simulink model "FMS"  (R2018b)
settings: configuration reference "FMS_config" (kept outside this file)
values from neighbouring files (symbols this model uses):
  FMS_EXPORT = Simulink.Parameter(FMS_EXPORT_VALUE)    [base_fms_init.m]    (also in base_fms_var.m; fms_model_init.m)
  FMS_PARAM = Simulink.Parameter(FMS_PARAM_VALUE)    [base_fms_init.m]    (also in base_fms_var.m; fms_model_init.m)
undefined symbols (not defined in the file or in its folder): actuator_cmd, DiscIntNeverNeededParam, mode, p_cmd, phi_cmd, psi_rate_cmd, q_cmd, r_cmd, reset, state, theta_cmd, throttle_cmd, timestamp, u_cmd, v_cmd, w_cmd
libraries: simulink x31, Rotation x2, Filter x2
(part 1 of 2)
settings Model: Creator=zouji  LastModifiedBy=zouji
settings ConfigSetRef: SourceLocation=Base Workspace

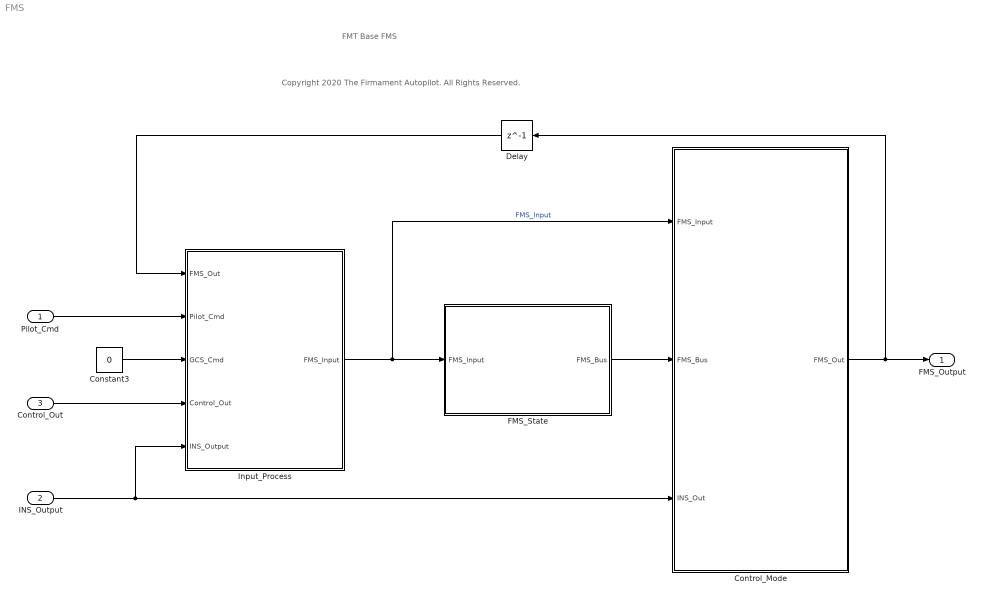
== system FMS ==
  note: FMT Base FMS
  note: Copyright 2020 The Firmament Autopilot. All Rights Reserved.
  Pilot_Cmd : Inport  OutDataTypeStr=Bus: Pilot_Cmd_Bus
  INS_Output : Inport  Port=2  OutDataTypeStr=Bus: INS_Out_Bus
  Control_Out : Inport  Port=3  OutDataTypeStr=Bus: Control_Out_Bus
  Constant3 : Constant  Value=0
  Control_Mode : Subsystem  TreatAsAtomicUnit=on
  Delay : Delay  DelayLength=1
  FMS_State : Subsystem  TreatAsAtomicUnit=on
  Input_Process : Subsystem  TreatAsAtomicUnit=on
  FMS_Output : Outport  OutDataTypeStr=Bus: FMS_Out_Bus
  wires:
  Control_Mode/1(FMS_Out) -> FMS_Output/1, Delay/1
  INS_Output/1 -> Input_Process/5(INS_Output), Control_Mode/3(INS_Out)
  Pilot_Cmd/1 -> Input_Process/2(Pilot_Cmd)
  Constant3/1 -> Input_Process/3(GCS_Cmd)
  Input_Process/1(FMS_Input) -> Control_Mode/1(FMS_Input), FMS_State/1(FMS_Input)  "FMS_Input"
  FMS_State/1(FMS_Bus) -> Control_Mode/2(FMS_Bus)
  Delay/1 -> Input_Process/1(FMS_Out)
  Control_Out/1 -> Input_Process/4(Control_Out)

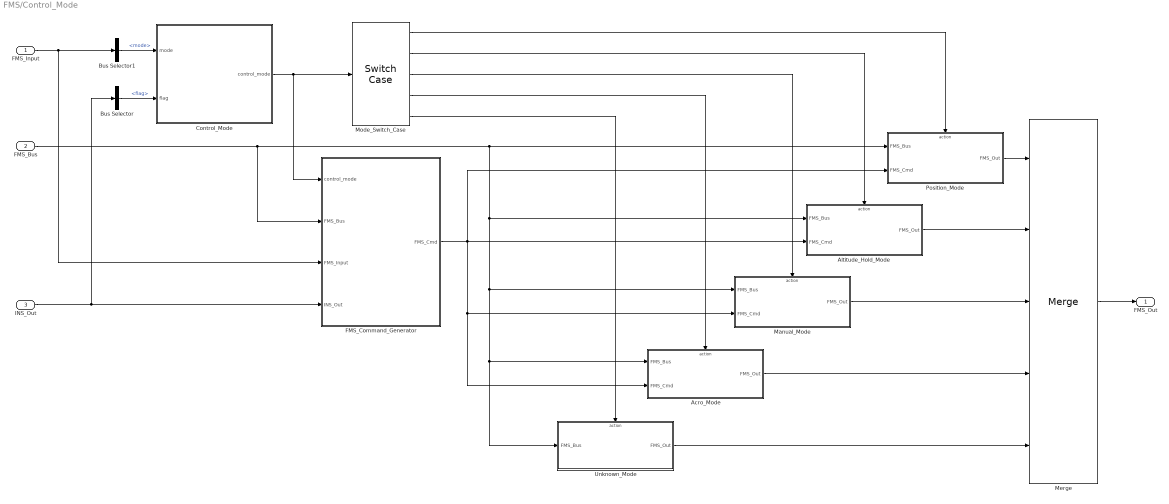
== system FMS/Control_Mode ==
  FMS_Input : Inport
  FMS_Bus : Inport  Port=2
  INS_Out : Inport  Port=3
  Acro_Mode : Subsystem  TreatAsAtomicUnit=on
  Altitude_Hold_Mode : Subsystem  TreatAsAtomicUnit=on
  Bus Selector : BusSelector  OutputSignals=flag
  Bus Selector1 : BusSelector  OutputSignals=stick_val.mode
  Control_Mode : Stateflow chart  TreatAsAtomicUnit=on
  FMS_Command_Generator : Subsystem
  Manual_Mode : Subsystem  TreatAsAtomicUnit=on
  Merge : Merge  Inputs=5
  Mode_Switch_Case : SwitchCase  CaseConditions={2,3,4,5}
  Position_Mode : Subsystem  TreatAsAtomicUnit=on
  Unknown_Mode : Subsystem  TreatAsAtomicUnit=on
  FMS_Out : Outport
  wires:
  INS_Out/1 -> Bus Selector/1, FMS_Command_Generator/4(INS_Out)
  FMS_Input/1 -> FMS_Command_Generator/3(FMS_Input), Bus Selector1/1
  Mode_Switch_Case/1 -> Position_Mode/Action
  Position_Mode/1(FMS_Out) -> Merge/1
  Mode_Switch_Case/5 -> Unknown_Mode/Action
  Bus Selector/1 -> Control_Mode/2(flag)  "<flag>"
  Merge/1 -> FMS_Out/1
  Unknown_Mode/1(FMS_Out) -> Merge/5
  FMS_Bus/1 -> Position_Mode/1(FMS_Bus), Unknown_Mode/1(FMS_Bus), Acro_Mode/1(FMS_Bus), Manual_Mode/1(FMS_Bus), Altitude_Hold_Mode/1(FMS_Bus), FMS_Command_Generator/2(FMS_Bus)
  Bus Selector1/1 -> Control_Mode/1(mode)  "<mode>"
  Control_Mode/1(control_mode) -> Mode_Switch_Case/1, FMS_Command_Generator/1(control_mode)
  Mode_Switch_Case/2 -> Altitude_Hold_Mode/Action
  Altitude_Hold_Mode/1(FMS_Out) -> Merge/2
  Mode_Switch_Case/3 -> Manual_Mode/Action
  Manual_Mode/1(FMS_Out) -> Merge/3
  Acro_Mode/1(FMS_Out) -> Merge/4
  Mode_Switch_Case/4 -> Acro_Mode/Action
  FMS_Command_Generator/1(FMS_Cmd) -> Acro_Mode/2(FMS_Cmd), Manual_Mode/2(FMS_Cmd), Altitude_Hold_Mode/2(FMS_Cmd), Position_Mode/2(FMS_Cmd)

== system FMS/FMS_State ==
  FMS_Input : Inport
  Bus Assignment : BusAssignment  AssignedSignals=actuator_cmd,state,reset,timestamp
  Bus Selector : BusSelector  OutputSignals=stick_val.stick_throttle_raw,event_cmd.arm_event,event_cmd.disarm_event,event_cmd.force_disarm_event,state_cmd.test_motor_state
  Compare To Constant : simulink/Logic and Bit Operations/Compare To Constant  relop=<  const=2  OutDataTypeStr=uint8
  Constant : Constant  Value=0  OutDataTypeStr=Bus: FMS_Out_Bus
  State_Management : Stateflow chart  TreatAsAtomicUnit=on
  expand_pwm : Subsystem
  timestamp : Subsystem  mask{sample_time=FMS_EXPORT.period}
      mask prompts: sample_time "sample time (ms)"
  FMS_Bus : Outport
  wires:
  Constant/1 -> Bus Assignment/1
  Bus Assignment/1 -> FMS_Bus/1
  FMS_Input/1 -> Bus Selector/1
  State_Management/1(PWM_Cmd) -> expand_pwm/1(pwm_in)
  expand_pwm/1(pwm_out) -> Bus Assignment/2
  Compare To Constant/1 -> Bus Assignment/4
  timestamp/1(timestamp_ms) -> Bus Assignment/5
  Bus Selector/1 -> State_Management/1(stick_throttle)  "<stick_throttle_raw>"
  Bus Selector/2 -> State_Management/2(arm_event)  "<arm_event>"
  Bus Selector/3 -> State_Management/3(disarm_event)  "<disarm_event>"
  Bus Selector/4 -> State_Management/4(force_disarm_event)  "<force_disarm_event>"
  Bus Selector/5 -> State_Management/5(test_motor_state)  "<test_motor_state>"
  State_Management/2(State) -> Compare To Constant/1, Bus Assignment/3

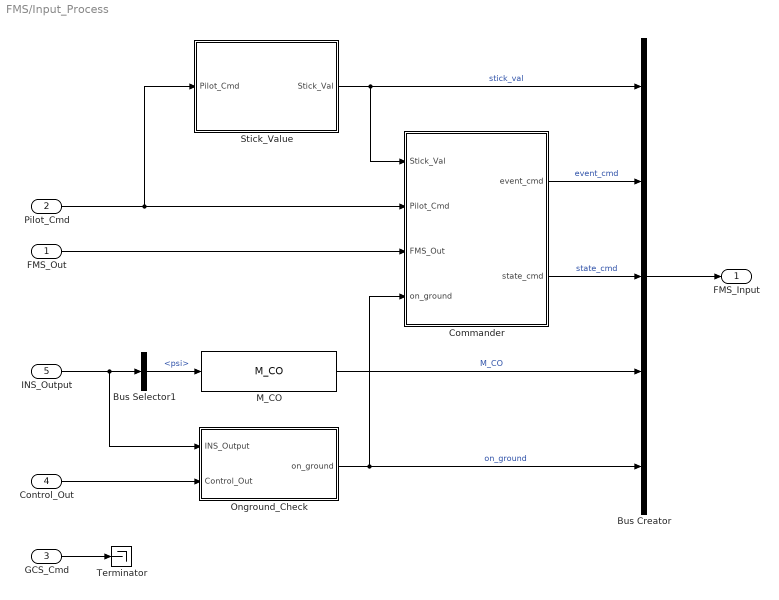
== system FMS/Input_Process ==
  FMS_Out : Inport
  Pilot_Cmd : Inport  Port=2
  GCS_Cmd : Inport  Port=3
  Control_Out : Inport  Port=4
  INS_Output : Inport  Port=5
  Bus Creator : BusCreator  Inputs=5
  Bus Selector1 : BusSelector  OutputSignals=psi
  Commander : Subsystem
  M_CO : Rotation/M_CO  SystemSampleTime=-1
  Onground_Check : Subsystem
  Stick_Value : Subsystem
  Terminator : Terminator
  FMS_Input : Outport
  wires:
  GCS_Cmd/1 -> Terminator/1
  Pilot_Cmd/1 -> Stick_Value/1(Pilot_Cmd), Commander/2(Pilot_Cmd)
  Bus Creator/1 -> FMS_Input/1
  INS_Output/1 -> Onground_Check/1(INS_Output), Bus Selector1/1
  Bus Selector1/1 -> M_CO/1  "<psi>"
  M_CO/1 -> Bus Creator/4  "M_CO"
  Commander/1(event_cmd) -> Bus Creator/2  "event_cmd"
  Commander/2(state_cmd) -> Bus Creator/3  "state_cmd"
  Stick_Value/1(Stick_Val) -> Commander/1(Stick_Val), Bus Creator/1  "stick_val"
  FMS_Out/1 -> Commander/3(FMS_Out)
  Control_Out/1 -> Onground_Check/2(Control_Out)
  Onground_Check/1(on_ground) -> Commander/4(on_ground), Bus Creator/5  "on_ground"

== system FMS/Control_Mode/Acro_Mode ==
  FMS_Bus : Inport
  FMS_Cmd : Inport  Port=2
  Action Port : ActionPort  InitializeStates=reset  ActionType=case
  Bus Assignment : BusAssignment  AssignedSignals=mode,throttle_cmd,p_cmd,q_cmd,r_cmd
  Bus Selector : BusSelector  OutputSignals=throttle_cmd,p_cmd,q_cmd,r_cmd
  Constant : Constant  Value=5  OutDataTypeStr=Inherit: Inherit via back propagation
  FMS_Out : Outport
  wires:
  Bus Assignment/1 -> FMS_Out/1
  Constant/1 -> Bus Assignment/2
  FMS_Bus/1 -> Bus Assignment/1
  Bus Selector/1 -> Bus Assignment/3  "<throttle_cmd>"
  Bus Selector/2 -> Bus Assignment/4  "<p_cmd>"
  Bus Selector/3 -> Bus Assignment/5  "<q_cmd>"
  Bus Selector/4 -> Bus Assignment/6  "<r_cmd>"
  FMS_Cmd/1 -> Bus Selector/1

== system FMS/Control_Mode/Altitude_Hold_Mode ==
  FMS_Bus : Inport
  FMS_Cmd : Inport  Port=2
  Action Port : ActionPort  InitializeStates=reset  ActionType=case
  Bus Assignment : BusAssignment  AssignedSignals=mode,phi_cmd,theta_cmd,w_cmd,psi_rate_cmd
  Bus Selector : BusSelector  OutputSignals=phi_cmd,thera_cmd,w_cmd,psi_rate_cmd
  alt_hold_mode : Constant  Value=3  OutDataTypeStr=Inherit: Inherit via back propagation
  FMS_Out : Outport
  wires:
  FMS_Bus/1 -> Bus Assignment/1
  alt_hold_mode/1 -> Bus Assignment/2
  FMS_Cmd/1 -> Bus Selector/1
  Bus Assignment/1 -> FMS_Out/1
  Bus Selector/3 -> Bus Assignment/5  "<w_cmd>"
  Bus Selector/4 -> Bus Assignment/6  "<psi_rate_cmd>"
  Bus Selector/1 -> Bus Assignment/3  "<phi_cmd>"
  Bus Selector/2 -> Bus Assignment/4  "<thera_cmd>"

== system FMS/Control_Mode/FMS_Command_Generator ==
  control_mode : Inport
  FMS_Bus : Inport  Port=2
  FMS_Input : Inport  Port=3
  INS_Out : Inport  Port=4
  Angel_Rate_Command : Subsystem
  Attitude_Command : Subsystem
  Bus Creator : BusCreator  Inputs=10
  Psi_Rate_Command : Subsystem
  Throttle_Command : Subsystem
  Velocity_Command : Subsystem
  FMS_Cmd : Outport
  wires:
  FMS_Input/1 -> Attitude_Command/1(FMS_Input), Velocity_Command/2(FMS_Input), Throttle_Command/1(FMS_Input), Angel_Rate_Command/1(FMS_Input), Psi_Rate_Command/1(FMS_Input)
  INS_Out/1 -> Psi_Rate_Command/2(INS_Out), Velocity_Command/3(INS_Out)
  FMS_Bus/1 -> Psi_Rate_Command/3(FMS_Bus), Velocity_Command/4(FMS_Bus)
  Attitude_Command/1(phi_cmd_rad) -> Bus Creator/1  "phi_cmd"
  Attitude_Command/2(theta_cmd_rad) -> Bus Creator/2  "thera_cmd"
  Psi_Rate_Command/1(psi_rate_cmd_radPs) -> Bus Creator/3  "psi_rate_cmd"
  Velocity_Command/1(vel_u_cmd_C_mPs) -> Bus Creator/4  "u_cmd"
  Velocity_Command/2(vel_v_cmd_C_mPs) -> Bus Creator/5  "v_cmd"
  Velocity_Command/3(vel_w_cmd_C_mPs) -> Bus Creator/6  "w_cmd"
  Throttle_Command/1(throttle_cmd) -> Bus Creator/7  "throttle_cmd"
  Angel_Rate_Command/1(p_cmd_radPs) -> Bus Creator/8  "p_cmd"
  Angel_Rate_Command/2(q_cmd_radPs) -> Bus Creator/9  "q_cmd"
  Angel_Rate_Command/3(r_cmd_radPs) -> Bus Creator/10  "r_cmd"
  Bus Creator/1 -> FMS_Cmd/1
  control_mode/1 -> Velocity_Command/1(control_mode), Psi_Rate_Command/4(control_mode)

== system FMS/Control_Mode/Manual_Mode ==
  FMS_Bus : Inport
  FMS_Cmd : Inport  Port=2
  Action Port : ActionPort  InitializeStates=reset  ActionType=case
  Bus Assignment : BusAssignment  AssignedSignals=mode,throttle_cmd,phi_cmd,theta_cmd,psi_rate_cmd
  Bus Selector : BusSelector  OutputSignals=throttle_cmd,phi_cmd,thera_cmd,psi_rate_cmd
  manual_mode : Constant  Value=4  OutDataTypeStr=Inherit: Inherit via back propagation
  FMS_Out : Outport
  wires:
  Bus Assignment/1 -> FMS_Out/1
  FMS_Cmd/1 -> Bus Selector/1
  manual_mode/1 -> Bus Assignment/2
  FMS_Bus/1 -> Bus Assignment/1
  Bus Selector/1 -> Bus Assignment/3  "<throttle_cmd>"
  Bus Selector/2 -> Bus Assignment/4  "<phi_cmd>"
  Bus Selector/3 -> Bus Assignment/5  "<thera_cmd>"
  Bus Selector/4 -> Bus Assignment/6  "<psi_rate_cmd>"

== system FMS/Control_Mode/Position_Mode ==
  FMS_Bus : Inport
  FMS_Cmd : Inport  Port=2
  Action Port : ActionPort  InitializeStates=reset  ActionType=case
  Bus Assignment : BusAssignment  AssignedSignals=mode,u_cmd,v_cmd,w_cmd,psi_rate_cmd
  Bus Selector : BusSelector  OutputSignals=u_cmd,v_cmd,w_cmd,psi_rate_cmd
  position_mode : Constant  Value=2  OutDataTypeStr=Inherit: Inherit via back propagation
  FMS_Out : Outport
  wires:
  FMS_Bus/1 -> Bus Assignment/1
  position_mode/1 -> Bus Assignment/2
  Bus Assignment/1 -> FMS_Out/1
  Bus Selector/1 -> Bus Assignment/3  "<u_cmd>"
  Bus Selector/2 -> Bus Assignment/4  "<v_cmd>"
  Bus Selector/3 -> Bus Assignment/5  "<w_cmd>"
  Bus Selector/4 -> Bus Assignment/6  "<psi_rate_cmd>"
  FMS_Cmd/1 -> Bus Selector/1

== system FMS/Control_Mode/Unknown_Mode ==
  FMS_Bus : Inport
  Action Port : ActionPort  InitializeStates=reset  ActionType=default
  Bus Assignment : BusAssignment  AssignedSignals=mode,reset
  Constant1 : Constant  Value=0  OutDataTypeStr=Inherit: Inherit via back propagation
  Constant2 : Constant  OutDataTypeStr=Inherit: Inherit via back propagation
  FMS_Out : Outport
  wires:
  Bus Assignment/1 -> FMS_Out/1
  FMS_Bus/1 -> Bus Assignment/1
  Constant1/1 -> Bus Assignment/2
  Constant2/1 -> Bus Assignment/3

== system FMS/FMS_State/expand_pwm ==
  pwm_in : Inport
  Multiply : Product  OutDataTypeStr=uint16
  One : Constant  Value=ones(16,1)  OutDataTypeStr=uint16
  pwm_out : Outport
  wires:
  pwm_in/1 -> Multiply/2
  One/1 -> Multiply/1
  Multiply/1 -> pwm_out/1

== system FMS/FMS_State/timestamp ==
  Constant : Constant  Value=sample_time  OutDataTypeStr=uint32
  Data Type Conversion : DataTypeConversion  OutDataTypeStr=uint32
  Discrete-Time Integrator : DiscreteIntegrator  IntegratorMethod=Accumulation: Forward Euler  SampleTime=-1  ICPrevOutput=DiscIntNeverNeededParam  ICPrevScaledInput=DiscIntNeverNeededParam
  timestamp_ms : Outport
  wires:
  Discrete-Time Integrator/1 -> Data Type Conversion/1
  Constant/1 -> Discrete-Time Integrator/1
  Data Type Conversion/1 -> timestamp_ms/1

== system FMS/Input_Process/Commander ==
  Stick_Val : Inport
  Pilot_Cmd : Inport  Port=2
  FMS_Out : Inport  Port=3
  on_ground : Inport  Port=4
  Event_Commander : Subsystem
  State_Commander : Subsystem
  event_cmd : Outport
  state_cmd : Outport  Port=2
  wires:
  Pilot_Cmd/1 -> State_Commander/1(Pilot_Cmd), Event_Commander/3(Pilot_Cmd)
  Event_Commander/1(Event_Cmd) -> event_cmd/1
  FMS_Out/1 -> Event_Commander/2(FMS_Out)
  Stick_Val/1 -> Event_Commander/1(Stick_Val)
  on_ground/1 -> Event_Commander/4(on_ground)
  State_Commander/1(State_Cmd) -> state_cmd/1

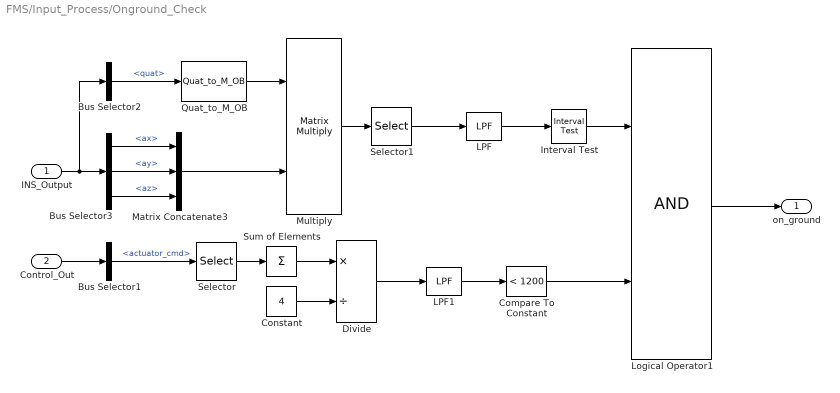
== system FMS/Input_Process/Onground_Check ==
  INS_Output : Inport
  Control_Out : Inport  Port=2
  Bus Selector1 : BusSelector  OutputSignals=actuator_cmd
  Bus Selector2 : BusSelector  OutputSignals=quat
  Bus Selector3 : BusSelector  OutputSignals=ax,ay,az
  Compare To Constant : simulink/Logic and Bit Operations/Compare To Constant  relop=<  const=1200  OutDataTypeStr=boolean
  Constant : Constant  Value=4  OutDataTypeStr=uint16
  Divide : Product  Inputs=*/
  Interval Test : simulink/Logic and Bit Operations/Interval Test  IntervalClosedRight=on  uplimit=single(-9.806+1)  IntervalClosedLeft=on  lowlimit=single(-9.806-1)  OutDataTypeStr=boolean
  LPF : Filter/LPF  T=0.5
  LPF1 : Filter/LPF  T=0.1
  Logical Operator1 : Logic  AllPortsSameDT=off  OutDataTypeStr=boolean
  Matrix Concatenate3 : Concatenate  NumInputs=3  ConcatenateDimension=2
  Multiply : Product  Multiplication=Matrix(*)
  Quat_to_M_OB : Rotation/Quat_to_M_OB  SystemSampleTime=-1
  Selector : Selector  InputPortWidth=16  IndexOptions=Index vector (dialog)  Indices=[1:4]  OutputSizes=1
  Selector1 : Selector  InputPortWidth=3  IndexOptions=Index vector (dialog)  Indices=3  OutputSizes=1
  Sum of Elements : Sum  Inputs=+
  on_ground : Outport
  wires:
  Multiply/1 -> Selector1/1
  Quat_to_M_OB/1 -> Multiply/1
  Bus Selector3/2 -> Matrix Concatenate3/2  "<ay>"
  Compare To Constant/1 -> Logical Operator1/2
  Bus Selector3/3 -> Matrix Concatenate3/3  "<az>"
  Matrix Concatenate3/1 -> Multiply/2
  Bus Selector1/1 -> Selector/1  "<actuator_cmd>"
  Bus Selector3/1 -> Matrix Concatenate3/1  "<ax>"
  Bus Selector2/1 -> Quat_to_M_OB/1  "<quat>"
  Selector/1 -> Sum of Elements/1
  INS_Output/1 -> Bus Selector2/1, Bus Selector3/1
  Logical Operator1/1 -> on_ground/1
  Control_Out/1 -> Bus Selector1/1
  Selector1/1 -> LPF/1
  Interval Test/1 -> Logical Operator1/1
  Sum of Elements/1 -> Divide/1
  Constant/1 -> Divide/2
  Divide/1 -> LPF1/1
  LPF/1 -> Interval Test/1
  LPF1/1 -> Compare To Constant/1

== system FMS/Input_Process/Stick_Value ==
  Pilot_Cmd : Inport
  Bus Creator : BusCreator  Inputs=9
  Bus Selector : BusSelector  OutputSignals=ls_lr,ls_ud,rs_lr,rs_ud,mode
  Dead_Zone : Subsystem  mask{len=FMS_PARAM.YAW_DZ}
      mask prompts: len "Zone Half Length"
  Dead_Zone1 : Subsystem  mask{len=FMS_PARAM.THROTTLE_DZ}
      mask prompts: len "Zone Half Length"
  Dead_Zone2 : Subsystem  mask{len=FMS_PARAM.ROLL_DZ}
      mask prompts: len "Zone Half Length"
  Dead_Zone3 : Subsystem  mask{len=FMS_PARAM.PITCH_DZ}
      mask prompts: len "Zone Half Length"
  Saturation{,1..3} (4 alike) : Saturate  UpperLimit=1  LowerLimit=-1
  Signal Copy4 : SignalConversion  OverrideOpt=off
  Stick_Val : Outport
  wires:
  Saturation/1 -> Bus Creator/2, Dead_Zone/1(in)  "stick_yaw_raw"
  Bus Selector/2 -> Saturation1/1  "<ls_ud>"
  Bus Selector/1 -> Saturation/1  "<ls_lr>"
  Saturation2/1 -> Bus Creator/6, Dead_Zone2/1(in)  "stick_roll_raw"
  Saturation1/1 -> Bus Creator/4, Dead_Zone1/1(in)  "stick_throttle_raw"
  Saturation3/1 -> Bus Creator/8, Dead_Zone3/1(in)  "stick_pitch_raw"
  Bus Selector/5 -> Signal Copy4/1  "<mode>"
  Bus Selector/3 -> Saturation2/1  "<rs_lr>"
  Bus Selector/4 -> Saturation3/1  "<rs_ud>"
  Dead_Zone/1(out) -> Bus Creator/1  "stick_yaw"
  Pilot_Cmd/1 -> Bus Selector/1
  Dead_Zone1/1(out) -> Bus Creator/3  "stick_throttle"
  Dead_Zone2/1(out) -> Bus Creator/5  "stick_roll"
  Dead_Zone3/1(out) -> Bus Creator/7  "stick_pitch"
  Signal Copy4/1 -> Bus Creator/9  "mode"
  Bus Creator/1 -> Stick_Val/1

== system FMS/Control_Mode/FMS_Command_Generator/Angel_Rate_Command ==
  FMS_Input : Inport
  Bus Selector : BusSelector  OutputSignals=stick_val.stick_roll_raw,stick_val.stick_pitch_raw,stick_val.stick_yaw_raw
  Gain : Gain  Gain=pi/3  OutDataTypeStr=Inherit: Same as input
  Gain1 : Gain  Gain=-pi/3  OutDataTypeStr=Inherit: Same as input
  Gain2 : Gain  Gain=pi/3  OutDataTypeStr=Inherit: Same as input
  p_cmd_radPs : Outport
  q_cmd_radPs : Outport  Port=2
  r_cmd_radPs : Outport  Port=3
  wires:
  Bus Selector/2 -> Gain1/1  "<stick_pitch_raw>"
  Bus Selector/1 -> Gain/1  "<stick_roll_raw>"
  FMS_Input/1 -> Bus Selector/1
  Gain/1 -> p_cmd_radPs/1
  Gain1/1 -> q_cmd_radPs/1
  Bus Selector/3 -> Gain2/1  "<stick_yaw_raw>"
  Gain2/1 -> r_cmd_radPs/1

== system FMS/Control_Mode/FMS_Command_Generator/Attitude_Command ==
  FMS_Input : Inport
  Bus Selector : BusSelector  OutputSignals=stick_val.stick_roll,stick_val.stick_pitch
  Gain : Gain  Gain=FMS_PARAM.ROLL_PITCH_LIM
  Gain1 : Gain  Gain=-FMS_PARAM.ROLL_PITCH_LIM
  Phi_CMD_TD : Subsystem
  Thera_CMD_TD : Subsystem
  phi_cmd_rad : Outport
  theta_cmd_rad : Outport  Port=2
  wires:
  Gain/1 -> Phi_CMD_TD/1(v)
  FMS_Input/1 -> Bus Selector/1
  Bus Selector/1 -> Gain/1  "<stick_roll>"
  Bus Selector/2 -> Gain1/1  "<stick_pitch>"
  Gain1/1 -> Thera_CMD_TD/1(v)
  Phi_CMD_TD/1(v1) -> phi_cmd_rad/1
  Thera_CMD_TD/1(v1) -> theta_cmd_rad/1

== system FMS/Control_Mode/FMS_Command_Generator/Psi_Rate_Command ==
  FMS_Input : Inport
  INS_Out : Inport  Port=2
  FMS_Bus : Inport  Port=3
  control_mode : Inport  Port=4
  Bus Selector : BusSelector  OutputSignals=state
  Motion_Check : Subsystem
  Psi_Rate_Commander : Subsystem
  Update : Subsystem
  psi_rate_cmd_radPs : Outport
  wires:
  INS_Out/1 -> Motion_Check/2(INS_Out), Psi_Rate_Commander/4(INS_Out)
  FMS_Input/1 -> Motion_Check/1(FMS_Input), Psi_Rate_Commander/2(FMS_Input)
  FMS_Bus/1 -> Bus Selector/1
  Motion_Check/1(psi_motion_state) -> Psi_Rate_Commander/3(motion_state), Update/3(motion_state)  "psi_motion_state"
  Psi_Rate_Commander/1(psi_rate_cmd_radPs) -> psi_rate_cmd_radPs/1
  Update/1(update) -> Psi_Rate_Commander/1(update)
  control_mode/1 -> Update/2(control_mode)
  Bus Selector/1 -> Update/1(state)  "<state>"

== system FMS/Control_Mode/FMS_Command_Generator/Throttle_Command ==
  FMS_Input : Inport
  Add : Sum
  Bus Selector : BusSelector  OutputSignals=stick_val.stick_throttle_raw
  Constant : Constant  OutDataTypeStr=single
  Constant1 : Constant  Value=1000  OutDataTypeStr=uint32
  Gain : Gain  Gain=500  OutDataTypeStr=uint32
  Saturation : Saturate  UpperLimit=2  LowerLimit=0
  Sum : Sum  Inputs=|++
  throttle_cmd : Outport
  wires:
  FMS_Input/1 -> Bus Selector/1
  Gain/1 -> Add/1
  Bus Selector/1 -> Sum/1  "<stick_throttle_raw>"
  Add/1 -> throttle_cmd/1
  Constant/1 -> Sum/2
  Sum/1 -> Saturation/1
  Constant1/1 -> Add/2
  Saturation/1 -> Gain/1

== system FMS/Control_Mode/FMS_Command_Generator/Velocity_Command ==
  control_mode : Inport
  FMS_Input : Inport  Port=2
  INS_Out : Inport  Port=3
  FMS_Bus : Inport  Port=4
  Bus Selector : BusSelector  OutputSignals=state
  Demux : Demux  Outputs=3
  Motion_Check : Subsystem
  Update : Subsystem
  Velocity_Commander : Subsystem
  vel_u_cmd_C_mPs : Outport
  vel_v_cmd_C_mPs : Outport  Port=2
  vel_w_cmd_C_mPs : Outport  Port=3
  wires:
  Velocity_Commander/1(vel_cmd_C_mPs) -> Demux/1
  FMS_Input/1 -> Motion_Check/1(FMS_Input), Velocity_Commander/1(FMS_Input)
  INS_Out/1 -> Motion_Check/2(INS_Out), Velocity_Commander/4(INS_Out)
  Motion_Check/1(pos_motion_state) -> Update/3(motion_state), Velocity_Commander/3(motion_state)  "pos_motion_state"
  Demux/1 -> vel_u_cmd_C_mPs/1
  Demux/2 -> vel_v_cmd_C_mPs/1
  Demux/3 -> vel_w_cmd_C_mPs/1
  FMS_Bus/1 -> Bus Selector/1
  control_mode/1 -> Update/1(control_mode)
  Bus Selector/1 -> Update/2(state)  "<state>"
  Update/1(update) -> Velocity_Commander/2(update)  "update_pos"

== system FMS/Input_Process/Commander/Event_Commander ==
  Stick_Val : Inport
  FMS_Out : Inport  Port=2
  Pilot_Cmd : Inport  Port=3
  on_ground : Inport  Port=4
  Arm_Disarm_Event : Subsystem
  Bus Creator : BusCreator  Inputs=3
  Bus Selector2 : BusSelector  OutputSignals=cmd_1
  Compare To Constant : simulink/Logic and Bit Operations/Compare To Constant  relop===  const=1000  OutDataTypeStr=boolean
  Detect Increase : simulink/Logic and Bit Operations/Detect Increase  vinit=0.0  OutDataTypeStr=boolean
  Event_Cmd : Outport
  wires:
  Pilot_Cmd/1 -> Bus Selector2/1
  Bus Selector2/1 -> Compare To Constant/1  "<cmd_1>"
  Compare To Constant/1 -> Detect Increase/1
  Detect Increase/1 -> Bus Creator/3  "force_disarm_event"
  Bus Creator/1 -> Event_Cmd/1
  FMS_Out/1 -> Arm_Disarm_Event/2(FMS_Out)
  Stick_Val/1 -> Arm_Disarm_Event/1(Stick_Val)
  on_ground/1 -> Arm_Disarm_Event/3(on_ground)
  Arm_Disarm_Event/1(arm_event) -> Bus Creator/1  "arm_event"
  Arm_Disarm_Event/2(disarm_event) -> Bus Creator/2  "disarm_event"

== system FMS/Input_Process/Commander/State_Commander ==
  Pilot_Cmd : Inport
  Bus Creator1 : BusCreator  Inputs=1
  Bus Selector1 : BusSelector  OutputSignals=cmd_2
  Compare To Constant3 : simulink/Logic and Bit Operations/Compare To Constant  relop===  const=2000  OutDataTypeStr=boolean
  State_Cmd : Outport
  wires:
  Bus Selector1/1 -> Compare To Constant3/1  "<cmd_2>"
  Compare To Constant3/1 -> Bus Creator1/1  "test_motor_state"
  Pilot_Cmd/1 -> Bus Selector1/1
  Bus Creator1/1 -> State_Cmd/1

== system FMS/Input_Process/Stick_Value/Dead_Zone ==
  in : Inport
  Add : Sum
  Constant : Constant  Value=len  OutDataTypeStr=single
  Dead Zone : DeadZone  LowerValue=-len  UpperValue=len  SaturateOnIntegerOverflow=on
  Multiply : Product
  Sign : Signum
  out : Outport
  wires:
  in/1 -> Dead Zone/1
  Dead Zone/1 -> Sign/1, Add/1
  Sign/1 -> Multiply/1
  Constant/1 -> Multiply/2
  Multiply/1 -> Add/2
  Add/1 -> out/1

== system FMS/Input_Process/Stick_Value/Dead_Zone1 ==
  in : Inport
  Add : Sum
  Constant : Constant  Value=len  OutDataTypeStr=single
  Dead Zone : DeadZone  LowerValue=-len  UpperValue=len  SaturateOnIntegerOverflow=on
  Multiply : Product
  Sign : Signum
  out : Outport
  wires:
  Add/1 -> out/1
  Multiply/1 -> Add/2
  Constant/1 -> Multiply/2
  Sign/1 -> Multiply/1
  Dead Zone/1 -> Add/1, Sign/1
  in/1 -> Dead Zone/1

== system FMS/Input_Process/Stick_Value/Dead_Zone2 ==
  in : Inport
  Add : Sum
  Constant : Constant  Value=len  OutDataTypeStr=single
  Dead Zone : DeadZone  LowerValue=-len  UpperValue=len  SaturateOnIntegerOverflow=on
  Multiply : Product
  Sign : Signum
  out : Outport
  wires:
  in/1 -> Dead Zone/1
  Dead Zone/1 -> Sign/1, Add/1
  Sign/1 -> Multiply/1
  Constant/1 -> Multiply/2
  Multiply/1 -> Add/2
  Add/1 -> out/1

== system FMS/Input_Process/Stick_Value/Dead_Zone3 ==
  in : Inport
  Add : Sum
  Constant : Constant  Value=len  OutDataTypeStr=single
  Dead Zone : DeadZone  LowerValue=-len  UpperValue=len  SaturateOnIntegerOverflow=on
  Multiply : Product
  Sign : Signum
  out : Outport
  wires:
  Add/1 -> out/1
  Multiply/1 -> Add/2
  Constant/1 -> Multiply/2
  Sign/1 -> Multiply/1
  Dead Zone/1 -> Add/1, Sign/1
  in/1 -> Dead Zone/1

== system FMS/Control_Mode/FMS_Command_Generator/Attitude_Command/Phi_CMD_TD ==
  v : Inport
  Integrator : DiscreteIntegrator  SampleTime=-1  ICPrevOutput=DiscIntNeverNeededParam  ICPrevScaledInput=DiscIntNeverNeededParam
  Integrator1 : DiscreteIntegrator  SampleTime=-1  ICPrevOutput=DiscIntNeverNeededParam  ICPrevScaledInput=DiscIntNeverNeededParam
  Subtract : Sum  Inputs=+-
  "fhan " : Subsystem  mask{r0=4*pi, h0=0.04}
      mask DialogControl ParameterGroupVar Prompt: fhan(v1,v2,r0,h0)
  v1 : Outport
  wires:
  Integrator1/1 -> v1/1, Subtract/1
  v/1 -> Subtract/2
  Integrator/1 -> "fhan "/2(v2), Integrator1/1  "v2"
  Subtract/1 -> "fhan "/1(v1)
  "fhan "/1(fhan) -> Integrator/1

== system FMS/Control_Mode/FMS_Command_Generator/Attitude_Command/Thera_CMD_TD ==
  v : Inport
  Integrator : DiscreteIntegrator  SampleTime=-1  ICPrevOutput=DiscIntNeverNeededParam  ICPrevScaledInput=DiscIntNeverNeededParam
  Integrator1 : DiscreteIntegrator  SampleTime=-1  ICPrevOutput=DiscIntNeverNeededParam  ICPrevScaledInput=DiscIntNeverNeededParam
  Subtract : Sum  Inputs=+-
  "fhan " : Subsystem  mask{r0=4*pi, h0=0.04}
      mask DialogControl ParameterGroupVar Prompt: fhan(v1,v2,r0,h0)
  v1 : Outport
  wires:
  "fhan "/1(fhan) -> Integrator/1
  Subtract/1 -> "fhan "/1(v1)
  Integrator/1 -> "fhan "/2(v2), Integrator1/1  "v2"
  v/1 -> Subtract/2
  Integrator1/1 -> Subtract/1, v1/1

== system FMS/Control_Mode/FMS_Command_Generator/Psi_Rate_Command/Motion_Check ==
  FMS_Input : Inport
  INS_Out : Inport  Port=2
  Motion_State : Stateflow chart  TreatAsAtomicUnit=on
  heading_rate : Subsystem
  move_check : Subsystem
  psi_motion_state : Outport
  wires:
  heading_rate/1(heading_rate) -> Motion_State/2(heading_rate)
  Motion_State/1(state) -> psi_motion_state/1
  FMS_Input/1 -> move_check/1(FMS_Input)
  move_check/1(move_request) -> Motion_State/1(move_cmd)
  INS_Out/1 -> heading_rate/1(INS_Out)

== system FMS/Control_Mode/FMS_Command_Generator/Psi_Rate_Command/Psi_Rate_Commander ==
  update : Inport
  FMS_Input : Inport  Port=2
  motion_state : Inport  Port=3
  INS_Out : Inport  Port=4
  Compare To Constant : simulink/Logic and Bit Operations/Compare To Constant  relop===  const=2  OutDataTypeStr=boolean
  Heading_Control : Subsystem
  Motion_Heading_Rate : Subsystem
  Saturation : Saturate  UpperLimit=FMS_PARAM.YAW_RATE_LIM  LowerLimit=-FMS_PARAM.YAW_RATE_LIM
  Switch : Switch  Criteria=u2 > Threshold
  TD : Subsystem
  psi_rate_cmd_radPs : Outport
  wires:
  Compare To Constant/1 -> Switch/2
  motion_state/1 -> Motion_Heading_Rate/1(motion_state), Compare To Constant/1
  Heading_Control/1(psi_rate_cmd_radPs) -> Switch/1
  Motion_Heading_Rate/1(psi_rate_cmd_radPs) -> Switch/3
  INS_Out/1 -> Heading_Control/2(INS_Out)
  FMS_Input/1 -> Motion_Heading_Rate/2(FMS_Input)
  Switch/1 -> Saturation/1
  Saturation/1 -> TD/1(v)
  TD/1(v1) -> psi_rate_cmd_radPs/1
  update/1 -> Heading_Control/1(update)

== system FMS/Control_Mode/FMS_Command_Generator/Psi_Rate_Command/Update ==
  state : Inport
  control_mode : Inport  Port=2
  motion_state : Inport  Port=3
  Compare To Constant1 : simulink/Logic and Bit Operations/Compare To Constant  relop=>=  const=1  OutDataTypeStr=boolean
  Compare To Constant2 : simulink/Logic and Bit Operations/Compare To Constant  relop=<=  const=4  OutDataTypeStr=boolean
  Compare To Constant3 : simulink/Logic and Bit Operations/Compare To Constant  relop===  const=2  OutDataTypeStr=boolean
  Compare To Constant4 : simulink/Logic and Bit Operations/Compare To Constant  relop===  const=2  OutDataTypeStr=boolean
  Detect Increase1 : simulink/Logic and Bit Operations/Detect Increase  vinit=0.0  OutDataTypeStr=boolean
  Detect Increase2 : simulink/Logic and Bit Operations/Detect Increase  vinit=0.0  OutDataTypeStr=boolean
  Detect Increase3 : simulink/Logic and Bit Operations/Detect Increase  vinit=0.0  OutDataTypeStr=boolean
  Logical Operator1 : Logic  Operator=OR  Inputs=3  AllPortsSameDT=off  OutDataTypeStr=boolean
  Logical Operator2 : Logic  Operator=OR  AllPortsSameDT=off  OutDataTypeStr=boolean
  update : Outport
  wires:
  state/1 -> Compare To Constant3/1
  Compare To Constant4/1 -> Detect Increase3/1
  Compare To Constant3/1 -> Detect Increase2/1
  Detect Increase2/1 -> Logical Operator1/2
  motion_state/1 -> Compare To Constant4/1
  Logical Operator1/1 -> update/1
  Detect Increase3/1 -> Logical Operator1/1
  control_mode/1 -> Compare To Constant2/1, Compare To Constant1/1
  Compare To Constant1/1 -> Logical Operator2/1
  Compare To Constant2/1 -> Logical Operator2/2
  Logical Operator2/1 -> Detect Increase1/1
  Detect Increase1/1 -> Logical Operator1/3

== system FMS/Control_Mode/FMS_Command_Generator/Velocity_Command/Motion_Check ==
  FMS_Input : Inport
  INS_Out : Inport  Port=2
  Motion_State : Subsystem
  line_speed : Subsystem
  move_check : Subsystem
  pos_motion_state : Outport
  wires:
  INS_Out/1 -> line_speed/1(INS_Out)
  move_check/1(move_request) -> Motion_State/1(move_request)
  Motion_State/1(pos_motion_state) -> pos_motion_state/1
  FMS_Input/1 -> move_check/1(FMS_Input)
  line_speed/1(line_speed) -> Motion_State/2(line_speed)

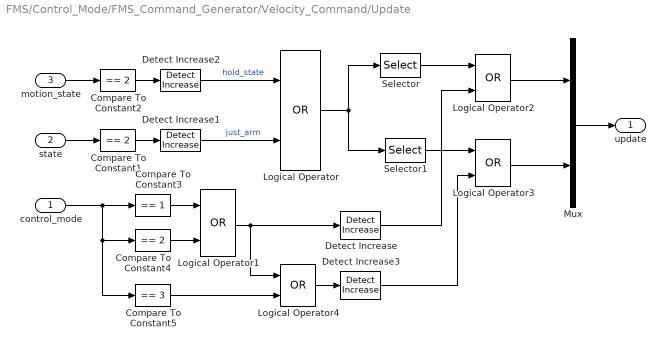
== system FMS/Control_Mode/FMS_Command_Generator/Velocity_Command/Update ==
  control_mode : Inport
  state : Inport  Port=2
  motion_state : Inport  Port=3
  Compare To Constant1 : simulink/Logic and Bit Operations/Compare To Constant  relop===  const=2  OutDataTypeStr=boolean
  Compare To Constant2 : simulink/Logic and Bit Operations/Compare To Constant  relop===  const=2  OutDataTypeStr=boolean
  Compare To Constant3 : simulink/Logic and Bit Operations/Compare To Constant  relop===  const=1  OutDataTypeStr=boolean
  Compare To Constant4 : simulink/Logic and Bit Operations/Compare To Constant  relop===  const=2  OutDataTypeStr=boolean
  Compare To Constant5 : simulink/Logic and Bit Operations/Compare To Constant  relop===  const=3  OutDataTypeStr=boolean
  Detect Increase{,1..3} (4 alike) : simulink/Logic and Bit Operations/Detect Increase  vinit=0.0  OutDataTypeStr=boolean
  Logical Operator{,1..4} (5 alike) : Logic  Operator=OR  AllPortsSameDT=off  OutDataTypeStr=boolean
  Mux : Mux  Inputs=2
  Selector : Selector  InputPortWidth=2  IndexOptions=Index vector (dialog)  Indices=1  OutputSizes=1
  Selector1 : Selector  InputPortWidth=2  IndexOptions=Index vector (dialog)  Indices=2  OutputSizes=1
  update : Outport
  wires:
  Compare To Constant3/1 -> Logical Operator1/1
  Compare To Constant4/1 -> Logical Operator1/2
  control_mode/1 -> Compare To Constant3/1, Compare To Constant4/1, Compare To Constant5/1
  Compare To Constant2/1 -> Detect Increase2/1
  Detect Increase2/1 -> Logical Operator/1  "hold_state"
  Logical Operator1/1 -> Logical Operator4/1, Detect Increase/1
  Detect Increase1/1 -> Logical Operator/2  "just_arm"
  motion_state/1 -> Compare To Constant2/1
  Compare To Constant1/1 -> Detect Increase1/1
  state/1 -> Compare To Constant1/1
  Logical Operator/1 -> Selector1/1, Selector/1
  Selector/1 -> Logical Operator2/1
  Detect Increase/1 -> Logical Operator2/2
  Selector1/1 -> Logical Operator3/1
  Compare To Constant5/1 -> Logical Operator4/2
  Detect Increase3/1 -> Logical Operator3/2
  Logical Operator2/1 -> Mux/1
  Logical Operator3/1 -> Mux/2
  Mux/1 -> update/1
  Logical Operator4/1 -> Detect Increase3/1

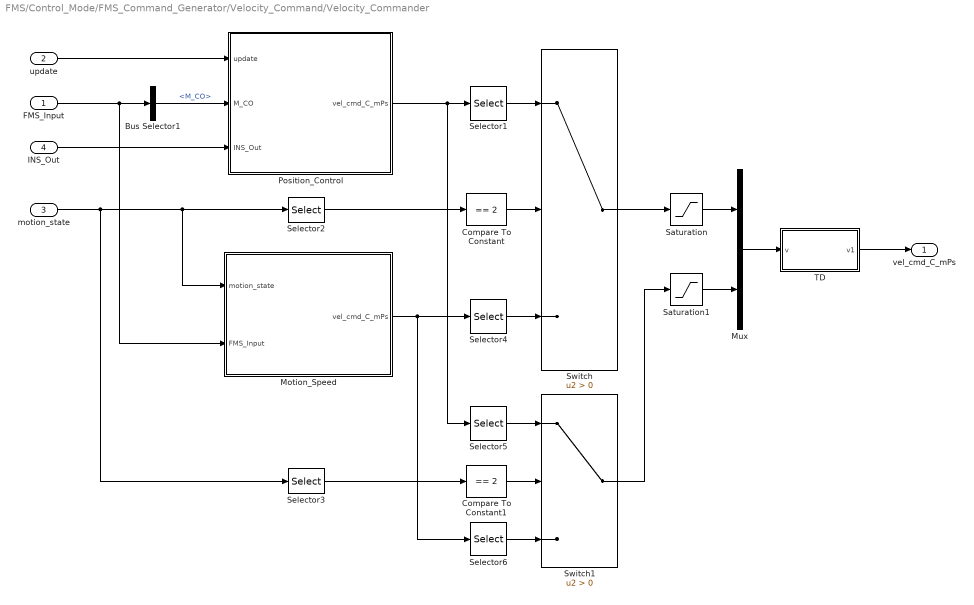
== system FMS/Control_Mode/FMS_Command_Generator/Velocity_Command/Velocity_Commander ==
  FMS_Input : Inport
  update : Inport  Port=2
  motion_state : Inport  Port=3
  INS_Out : Inport  Port=4
  Bus Selector1 : BusSelector  OutputSignals=M_CO
  Compare To Constant : simulink/Logic and Bit Operations/Compare To Constant  relop===  const=2  OutDataTypeStr=boolean
  Compare To Constant1 : simulink/Logic and Bit Operations/Compare To Constant  relop===  const=2  OutDataTypeStr=boolean
  Motion_Speed : Subsystem
  Mux : Mux  Inputs=2
  Position_Control : Subsystem
  Saturation : Saturate  UpperLimit=FMS_PARAM.VEL_XY_LIM  LowerLimit=-FMS_PARAM.VEL_XY_LIM
  Saturation1 : Saturate  UpperLimit=FMS_PARAM.VEL_Z_LIM  LowerLimit=-FMS_PARAM.VEL_Z_LIM
  Selector1 : Selector  InputPortWidth=3  IndexOptions=Index vector (dialog)  Indices=[1 2]  OutputSizes=1
  Selector2 : Selector  InputPortWidth=2  IndexOptions=Index vector (dialog)  Indices=1  OutputSizes=1
  Selector3 : Selector  InputPortWidth=2  IndexOptions=Index vector (dialog)  Indices=2  OutputSizes=1
  Selector4 : Selector  InputPortWidth=3  IndexOptions=Index vector (dialog)  Indices=[1 2]  OutputSizes=1
  Selector5 : Selector  InputPortWidth=3  IndexOptions=Index vector (dialog)  Indices=3  OutputSizes=1
  Selector6 : Selector  InputPortWidth=3  IndexOptions=Index vector (dialog)  Indices=3  OutputSizes=1
  Switch : Switch  Criteria=u2 > Threshold
  Switch1 : Switch  Criteria=u2 > Threshold
  TD : Subsystem
  vel_cmd_C_mPs : Outport
  wires:
  Motion_Speed/1(vel_cmd_C_mPs) -> Selector6/1, Selector4/1
  Position_Control/1(vel_cmd_C_mPs) -> Selector5/1, Selector1/1
  FMS_Input/1 -> Motion_Speed/2(FMS_Input), Bus Selector1/1
  Bus Selector1/1 -> Position_Control/2(M_CO)  "<M_CO>"
  INS_Out/1 -> Position_Control/3(INS_Out)
  Compare To Constant/1 -> Switch/2
  Mux/1 -> TD/1(v)
  Switch/1 -> Saturation/1
  Switch1/1 -> Saturation1/1
  motion_state/1 -> Motion_Speed/1(motion_state), Selector2/1, Selector3/1
  Selector3/1 -> Compare To Constant1/1
  Compare To Constant1/1 -> Switch1/2
  Selector1/1 -> Switch/1
  Selector4/1 -> Switch/3
  Selector6/1 -> Switch1/3
  Selector5/1 -> Switch1/1
  Selector2/1 -> Compare To Constant/1
  update/1 -> Position_Control/1(update)
  Saturation/1 -> Mux/1
  Saturation1/1 -> Mux/2
  TD/1(v1) -> vel_cmd_C_mPs/1

== system FMS/Input_Process/Commander/Event_Commander/Arm_Disarm_Event ==
  Stick_Val : Inport
  FMS_Out : Inport  Port=2
  on_ground : Inport  Port=3
  Arm_Event : Stateflow chart  TreatAsAtomicUnit=on
  Bus Selector : BusSelector  OutputSignals=stick_roll_raw,stick_pitch_raw,stick_throttle_raw
  Bus Selector1 : BusSelector  OutputSignals=state
  Disarm_Event : Stateflow chart  TreatAsAtomicUnit=on
  Logical Operator : Logic  AllPortsSameDT=off  OutDataTypeStr=boolean
  Logical Operator1 : Logic  AllPortsSameDT=off  OutDataTypeStr=boolean
  arm_allowed : Constant  OutDataTypeStr=uint8
  disarm_allowed : Constant  OutDataTypeStr=uint8
  arm_event : Outport
  disarm_event : Outport  Port=2
  wires:
  Arm_Event/1(arm_event) -> Logical Operator/1
  Stick_Val/1 -> Bus Selector/1
  Bus Selector/1 -> Arm_Event/1(stick_roll)  "<stick_roll_raw>"
  Bus Selector/2 -> Arm_Event/2(stick_pitch)  "<stick_pitch_raw>"
  Bus Selector/3 -> Arm_Event/3(stick_throttle)  "<stick_throttle_raw>"
  Disarm_Event/1(disarm_event) -> Logical Operator1/1
  on_ground/1 -> Disarm_Event/1(on_ground)
  FMS_Out/1 -> Bus Selector1/1
  Bus Selector1/1 -> Disarm_Event/2(state)  "<state>"
  Logical Operator/1 -> arm_event/1
  arm_allowed/1 -> Logical Operator/2
  disarm_allowed/1 -> Logical Operator1/2
  Logical Operator1/1 -> disarm_event/1

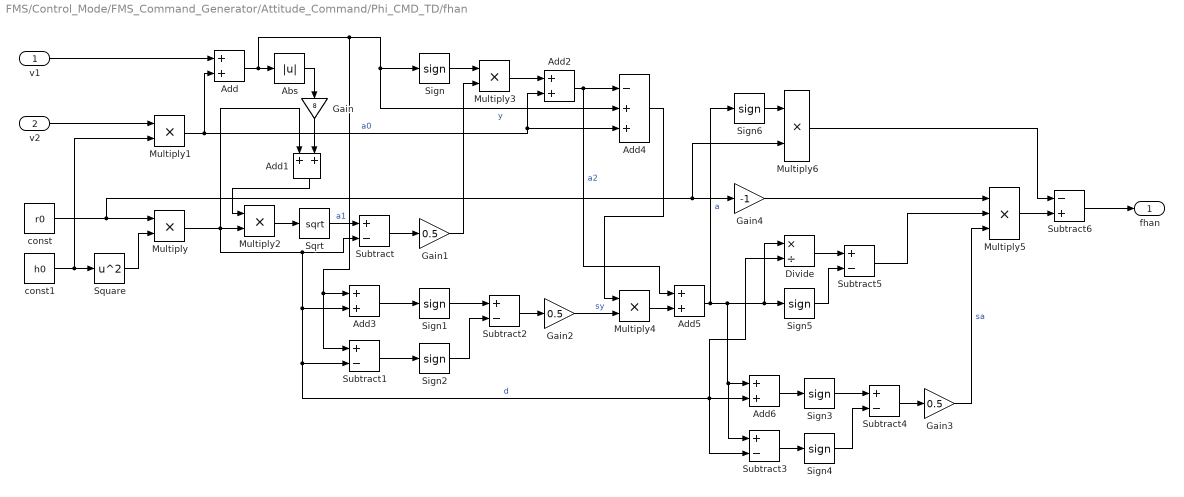
== system FMS/Control_Mode/FMS_Command_Generator/Attitude_Command/Phi_CMD_TD/fhan  ==
  v1 : Inport
  v2 : Inport  Port=2
  Abs : Abs
  Add{,1..3,5..6} (6 alike) : Sum  OutDataTypeStr=Inherit: Same as first input
  Add4 : Sum  Inputs=-++
  Divide : Product  Inputs=*/
  Gain : Gain  Gain=8
  Gain1 : Gain  Gain=0.5  OutDataTypeStr=Inherit: Same as input
  Gain2 : Gain  Gain=0.5  OutDataTypeStr=Inherit: Same as input
  Gain3 : Gain  Gain=0.5  OutDataTypeStr=Inherit: Same as input
  Gain4 : Gain  Gain=-1  OutDataTypeStr=Inherit: Same as input
  Multiply{,1..3} (4 alike) : Product  OutDataTypeStr=Inherit: Same as first input
  Multiply4 : Product  OutDataTypeStr=single
  Multiply5 : Product  Inputs=3
  Multiply6 : Product  OutDataTypeStr=single
  Sign{,1..6} (7 alike) : Signum
  Sqrt : Sqrt  SaturateOnIntegerOverflow=on
  Square : Math  Operator=square  SaturateOnIntegerOverflow=on
  Subtract{,1..5} (6 alike) : Sum  Inputs=+-  OutDataTypeStr=Inherit: Same as first input
  Subtract6 : Sum  Inputs=-+  OutDataTypeStr=Inherit: Same as first input
  const : Constant  Value=r0  OutDataTypeStr=single
  const1 : Constant  Value=h0  OutDataTypeStr=single
  fhan : Outport
  wires:
  Sign1/1 -> Subtract2/1
  Multiply2/1 -> Sqrt/1
  Square/1 -> Multiply/2
  Gain1/1 -> Multiply3/2
  Multiply6/1 -> Subtract6/1
  Multiply/1 -> Multiply2/2, Add1/1, Add3/2, Subtract1/2, Add6/2, Subtract3/2, Divide/2, Subtract/2  "d"
  Add6/1 -> Sign3/1
  Sign3/1 -> Subtract4/1
  Sign6/1 -> Multiply6/1
  Multiply5/1 -> Subtract6/2
  Gain4/1 -> Multiply5/1
  Subtract4/1 -> Gain3/1
  Add2/1 -> Add5/1, Add4/1  "a2"
  Subtract2/1 -> Gain2/1
  Add/1 -> Abs/1, Sign/1, Add4/2, Add3/1, Subtract1/1  "y"
  Multiply1/1 -> Add/2, Add2/2, Add4/3  "a0"
  Add5/1 -> Add6/1, Subtract3/1, Divide/1, Sign5/1, Sign6/1  "a"
  const1/1 -> Square/1, Multiply1/2
  Multiply4/1 -> Add5/2
  Subtract5/1 -> Multiply5/2
  Add3/1 -> Sign1/1
  const/1 -> Multiply/1, Gain4/1, Multiply6/2
  Gain/1 -> Add1/2
  Multiply3/1 -> Add2/1
  Divide/1 -> Subtract5/1
  Subtract1/1 -> Sign2/1
  Add1/1 -> Multiply2/1
  Subtract3/1 -> Sign4/1
  Sqrt/1 -> Subtract/1  "a1"
  Sign5/1 -> Subtract5/2
  Add4/1 -> Multiply4/1
  Abs/1 -> Gain/1
  Sign4/1 -> Subtract4/2
  Sign2/1 -> Subtract2/2
  Subtract6/1 -> fhan/1
  Subtract/1 -> Gain1/1
  Gain3/1 -> Multiply5/3  "sa"
  v2/1 -> Multiply1/1
  Gain2/1 -> Multiply4/2  "sy"
  Sign/1 -> Multiply3/1
  v1/1 -> Add/1

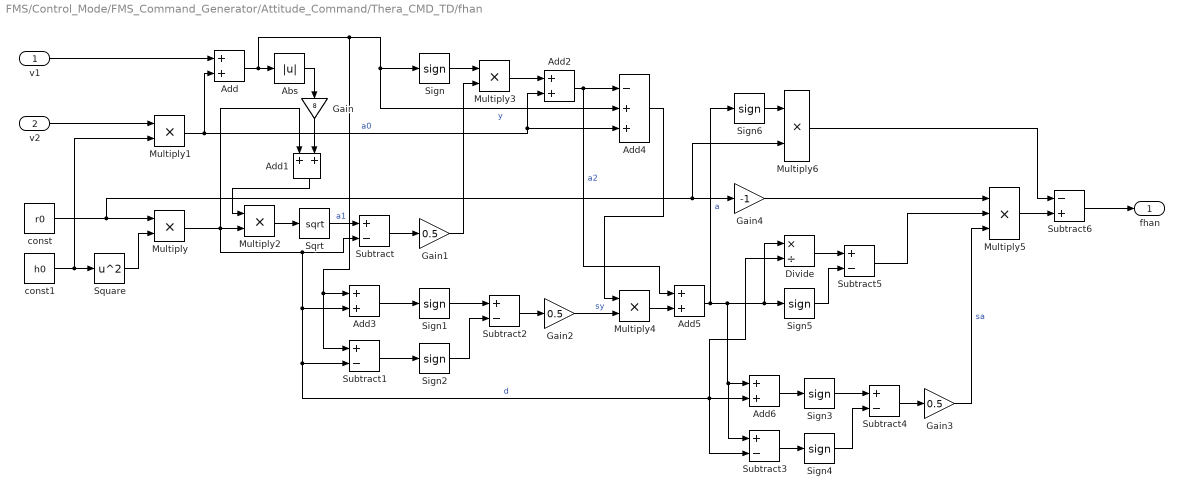
== system FMS/Control_Mode/FMS_Command_Generator/Attitude_Command/Thera_CMD_TD/fhan  ==
  v1 : Inport
  v2 : Inport  Port=2
  Abs : Abs
  Add{,1..3,5..6} (6 alike) : Sum  OutDataTypeStr=Inherit: Same as first input
  Add4 : Sum  Inputs=-++
  Divide : Product  Inputs=*/
  Gain : Gain  Gain=8
  Gain1 : Gain  Gain=0.5  OutDataTypeStr=Inherit: Same as input
  Gain2 : Gain  Gain=0.5  OutDataTypeStr=Inherit: Same as input
  Gain3 : Gain  Gain=0.5  OutDataTypeStr=Inherit: Same as input
  Gain4 : Gain  Gain=-1  OutDataTypeStr=Inherit: Same as input
  Multiply{,1..3} (4 alike) : Product  OutDataTypeStr=Inherit: Same as first input
  Multiply4 : Product  OutDataTypeStr=single
  Multiply5 : Product  Inputs=3
  Multiply6 : Product  OutDataTypeStr=single
  Sign{,1..6} (7 alike) : Signum
  Sqrt : Sqrt  SaturateOnIntegerOverflow=on
  Square : Math  Operator=square  SaturateOnIntegerOverflow=on
  Subtract{,1..5} (6 alike) : Sum  Inputs=+-  OutDataTypeStr=Inherit: Same as first input
  Subtract6 : Sum  Inputs=-+  OutDataTypeStr=Inherit: Same as first input
  const : Constant  Value=r0  OutDataTypeStr=single
  const1 : Constant  Value=h0  OutDataTypeStr=single
  fhan : Outport
  wires:
  Sign1/1 -> Subtract2/1
  Multiply2/1 -> Sqrt/1
  Square/1 -> Multiply/2
  Gain1/1 -> Multiply3/2
  Multiply6/1 -> Subtract6/1
  Multiply/1 -> Multiply2/2, Add1/1, Add3/2, Subtract1/2, Add6/2, Subtract3/2, Divide/2, Subtract/2  "d"
  Add6/1 -> Sign3/1
  Sign3/1 -> Subtract4/1
  Sign6/1 -> Multiply6/1
  Multiply5/1 -> Subtract6/2
  Gain4/1 -> Multiply5/1
  Subtract4/1 -> Gain3/1
  Add2/1 -> Add5/1, Add4/1  "a2"
  Subtract2/1 -> Gain2/1
  Add/1 -> Abs/1, Sign/1, Add4/2, Add3/1, Subtract1/1  "y"
  Multiply1/1 -> Add/2, Add2/2, Add4/3  "a0"
  Add5/1 -> Add6/1, Subtract3/1, Divide/1, Sign5/1, Sign6/1  "a"
  const1/1 -> Square/1, Multiply1/2
  Multiply4/1 -> Add5/2
  Subtract5/1 -> Multiply5/2
  Add3/1 -> Sign1/1
  const/1 -> Multiply/1, Gain4/1, Multiply6/2
  Gain/1 -> Add1/2
  Multiply3/1 -> Add2/1
  Divide/1 -> Subtract5/1
  Subtract1/1 -> Sign2/1
  Add1/1 -> Multiply2/1
  Subtract3/1 -> Sign4/1
  Sqrt/1 -> Subtract/1  "a1"
  Sign5/1 -> Subtract5/2
  Add4/1 -> Multiply4/1
  Abs/1 -> Gain/1
  Sign4/1 -> Subtract4/2
  Sign2/1 -> Subtract2/2
  Subtract6/1 -> fhan/1
  Subtract/1 -> Gain1/1
  Gain3/1 -> Multiply5/3  "sa"
  v2/1 -> Multiply1/1
  Gain2/1 -> Multiply4/2  "sy"
  Sign/1 -> Multiply3/1
  v1/1 -> Add/1

== system FMS/Control_Mode/FMS_Command_Generator/Psi_Rate_Command/Motion_Check/heading_rate ==
  note: TODO: Get the actual heading rate
  INS_Out : Inport
  Abs : Abs
  Bus Selector : BusSelector  OutputSignals=r
  heading_rate : Outport
  wires:
  INS_Out/1 -> Bus Selector/1
  Abs/1 -> heading_rate/1
  Bus Selector/1 -> Abs/1  "<r>"

== system FMS/Control_Mode/FMS_Command_Generator/Psi_Rate_Command/Motion_Check/move_check ==
  FMS_Input : Inport
  Bus Selector : BusSelector  OutputSignals=stick_val.stick_yaw
  Compare To Zero : simulink/Logic and Bit Operations/Compare To Zero  relop=~=  OutDataTypeStr=boolean
  move_request : Outport
  wires:
  FMS_Input/1 -> Bus Selector/1
  Compare To Zero/1 -> move_request/1
  Bus Selector/1 -> Compare To Zero/1  "<stick_yaw>"

== system FMS/Control_Mode/FMS_Command_Generator/Psi_Rate_Command/Psi_Rate_Commander/Heading_Control ==
  update : Inport
  INS_Out : Inport  Port=2
  Gain2 : Gain  Gain=FMS_PARAM.YAW_P  OutDataTypeStr=single
  Heading_Error : Subsystem
  psi_rate_cmd_radPs : Outport
  wires:
  INS_Out/1 -> Heading_Error/1(INS_Out)
  Heading_Error/1(psi_err_rad) -> Gain2/1
  Gain2/1 -> psi_rate_cmd_radPs/1
  update/1 -> Heading_Error/2(update)

== system FMS/Control_Mode/FMS_Command_Generator/Psi_Rate_Command/Psi_Rate_Commander/Motion_Heading_Rate ==
  motion_state : Inport
  FMS_Input : Inport  Port=2
  Bus Selector : BusSelector  OutputSignals=stick_val.stick_yaw
  Compare To Constant : simulink/Logic and Bit Operations/Compare To Constant  relop===  const=1  OutDataTypeStr=boolean
  Constant : Constant  Value=0  VectorParams1D=off  OutDataTypeStr=single
  Gain1 : Gain  Gain=FMS_PARAM.YAW_RATE_LIM  OutDataTypeStr=single
  Switch1 : Switch  Criteria=u2 > Threshold
  remap : Subsystem  mask{th=FMS_PARAM.YAW_DZ}
      mask prompts: th "Threshold"
  psi_rate_cmd_radPs : Outport
  wires:
  Constant/1 -> Switch1/1  "brake_speed"
  Switch1/1 -> psi_rate_cmd_radPs/1
  Gain1/1 -> Switch1/3
  motion_state/1 -> Compare To Constant/1
  Compare To Constant/1 -> Switch1/2  "is_braking"
  Bus Selector/1 -> remap/1(u)  "<stick_yaw>"
  remap/1(y) -> Gain1/1
  FMS_Input/1 -> Bus Selector/1

== system FMS/Control_Mode/FMS_Command_Generator/Psi_Rate_Command/Psi_Rate_Commander/TD ==
  v : Inport
  Integrator : DiscreteIntegrator  SampleTime=-1  ICPrevOutput=DiscIntNeverNeededParam  ICPrevScaledInput=DiscIntNeverNeededParam
  Integrator1 : DiscreteIntegrator  SampleTime=-1  ICPrevOutput=DiscIntNeverNeededParam  ICPrevScaledInput=DiscIntNeverNeededParam
  Subtract : Sum  Inputs=+-
  "fhan " : Subsystem  mask{r0=2*pi, h0=0.04}
      mask DialogControl ParameterGroupVar Prompt: fhan(v1,v2,r0,h0)
  v1 : Outport
  wires:
  Integrator1/1 -> v1/1, Subtract/1
  v/1 -> Subtract/2
  Integrator/1 -> "fhan "/2(v2), Integrator1/1  "v2"
  Subtract/1 -> "fhan "/1(v1)
  "fhan "/1(fhan) -> Integrator/1

== system FMS/Control_Mode/FMS_Command_Generator/Velocity_Command/Motion_Check/Motion_State ==
  move_request : Inport
  line_speed : Inport  Port=2
  Mux : Mux  Inputs=2
  Selector : Selector  InputPortWidth=2  IndexOptions=Index vector (dialog)  Indices=1  OutputSizes=1
  Selector1 : Selector  InputPortWidth=2  IndexOptions=Index vector (dialog)  Indices=1  OutputSizes=1
  Selector2 : Selector  InputPortWidth=2  IndexOptions=Index vector (dialog)  Indices=2  OutputSizes=1
  Selector3 : Selector  InputPortWidth=2  IndexOptions=Index vector (dialog)  Indices=2  OutputSizes=1
  XY_Motion_SM : Stateflow chart  TreatAsAtomicUnit=on
  Z_Motion_SM : Stateflow chart  TreatAsAtomicUnit=on
  pos_motion_state : Outport
  wires:
  move_request/1 -> Selector2/1, Selector/1
  XY_Motion_SM/1(state) -> Mux/1
  line_speed/1 -> Selector3/1, Selector1/1
  Selector/1 -> XY_Motion_SM/1(move_cmd)
  Selector1/1 -> XY_Motion_SM/2(speed)
  Selector2/1 -> Z_Motion_SM/1(move_cmd)
  Selector3/1 -> Z_Motion_SM/2(speed)
  Z_Motion_SM/1(state) -> Mux/2
  Mux/1 -> pos_motion_state/1

== system FMS/Control_Mode/FMS_Command_Generator/Velocity_Command/Motion_Check/line_speed ==
  INS_Out : Inport
  Abs : Abs
  Add : Sum
  Bus Selector : BusSelector  OutputSignals=vn,ve,vd
  Math Function : Math  Operator=square  SaturateOnIntegerOverflow=on
  Math Function1 : Math  Operator=square  SaturateOnIntegerOverflow=on
  Mux : Mux  Inputs=2
  Sqrt : Sqrt  SaturateOnIntegerOverflow=on
  line_speed : Outport
  wires:
  Add/1 -> Sqrt/1
  Math Function1/1 -> Add/2
  Math Function/1 -> Add/1
  Sqrt/1 -> Mux/1  "gnd_speed"
  Bus Selector/3 -> Abs/1  "<vd>"
  Bus Selector/2 -> Math Function1/1  "<ve>"
  Bus Selector/1 -> Math Function/1  "<vn>"
  INS_Out/1 -> Bus Selector/1
  Abs/1 -> Mux/2  "vz"
  Mux/1 -> line_speed/1

== system FMS/Control_Mode/FMS_Command_Generator/Velocity_Command/Motion_Check/move_check ==
  FMS_Input : Inport
  Bus Selector : BusSelector  OutputSignals=stick_val.stick_pitch,stick_val.stick_roll,stick_val.stick_throttle
  Compare To Zero1 : simulink/Logic and Bit Operations/Compare To Zero  relop=~=  OutDataTypeStr=boolean
  Compare To Zero2 : simulink/Logic and Bit Operations/Compare To Zero  relop=~=  OutDataTypeStr=boolean
  Logical Operator : Logic  Operator=OR  Inputs=1  AllPortsSameDT=off  OutDataTypeStr=boolean
  Mux : Mux  Inputs=2
  Mux1 : Mux  Inputs=2
  move_request : Outport
  wires:
  Mux1/1 -> Compare To Zero1/1
  Bus Selector/2 -> Mux1/2  "<stick_roll>"
  Bus Selector/1 -> Mux1/1  "<stick_pitch>"
  FMS_Input/1 -> Bus Selector/1
  Compare To Zero1/1 -> Logical Operator/1
  Logical Operator/1 -> Mux/1
  Bus Selector/3 -> Compare To Zero2/1  "<stick_throttle>"
  Compare To Zero2/1 -> Mux/2
  Mux/1 -> move_request/1

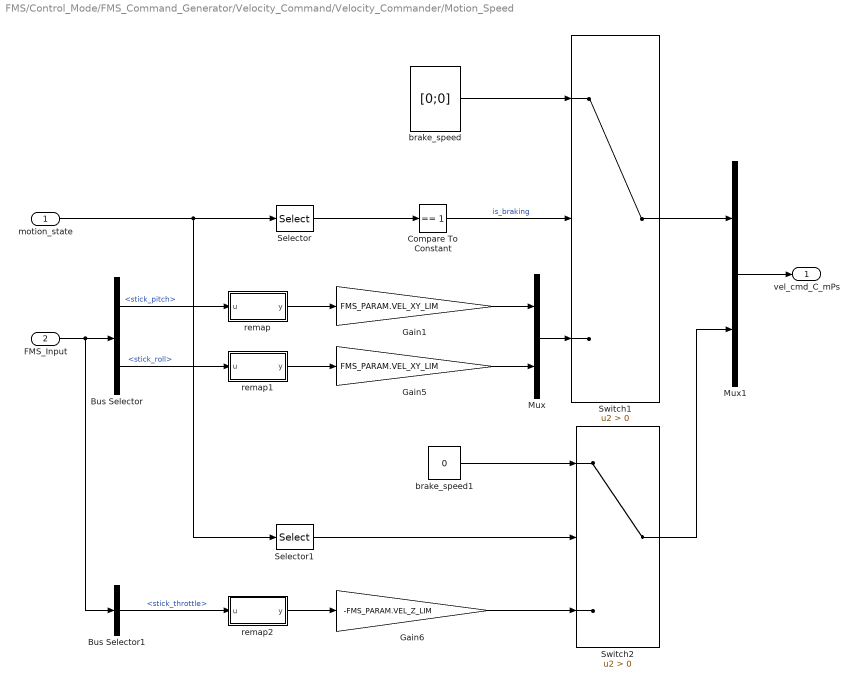
== system FMS/Control_Mode/FMS_Command_Generator/Velocity_Command/Velocity_Commander/Motion_Speed ==
  motion_state : Inport
  FMS_Input : Inport  Port=2
  Bus Selector : BusSelector  OutputSignals=stick_val.stick_pitch,stick_val.stick_roll
  Bus Selector1 : BusSelector  OutputSignals=stick_val.stick_throttle
  Compare To Constant : simulink/Logic and Bit Operations/Compare To Constant  relop===  const=1  OutDataTypeStr=boolean
  Gain1 : Gain  Gain=FMS_PARAM.VEL_XY_LIM  OutDataTypeStr=single
  Gain5 : Gain  Gain=FMS_PARAM.VEL_XY_LIM  OutDataTypeStr=single
  Gain6 : Gain  Gain=-FMS_PARAM.VEL_Z_LIM  OutDataTypeStr=single
  Mux : Mux  Inputs=2
  Mux1 : Mux  Inputs=2
  Selector : Selector  InputPortWidth=2  IndexOptions=Index vector (dialog)  Indices=1  OutputSizes=1
  Selector1 : Selector  InputPortWidth=2  IndexOptions=Index vector (dialog)  Indices=2  OutputSizes=1
  Switch1 : Switch  Criteria=u2 > Threshold
  Switch2 : Switch  Criteria=u2 > Threshold
  brake_speed : Constant  Value=[0;0]  VectorParams1D=off  OutDataTypeStr=single
  brake_speed1 : Constant  Value=0  VectorParams1D=off  OutDataTypeStr=single
  remap : Subsystem  mask{th=FMS_PARAM.PITCH_DZ}
      mask prompts: th "Threshold"
  remap1 : Subsystem  mask{th=FMS_PARAM.ROLL_DZ}
      mask prompts: th "Threshold"
  remap2 : Subsystem  mask{th=FMS_PARAM.THROTTLE_DZ}
      mask prompts: th "Threshold"
  vel_cmd_C_mPs : Outport
  wires:
  FMS_Input/1 -> Bus Selector/1, Bus Selector1/1
  motion_state/1 -> Selector1/1, Selector/1
  Bus Selector/1 -> remap/1(u)  "<stick_pitch>"
  Compare To Constant/1 -> Switch1/2  "is_braking"
  Gain1/1 -> Mux/1
  Bus Selector/2 -> remap1/1(u)  "<stick_roll>"
  Gain5/1 -> Mux/2
  Switch1/1 -> Mux1/1
  Mux/1 -> Switch1/3
  brake_speed/1 -> Switch1/1
  remap/1(y) -> Gain1/1
  remap1/1(y) -> Gain5/1
  remap2/1(y) -> Gain6/1
  Selector/1 -> Compare To Constant/1
  Selector1/1 -> Switch2/2
  Gain6/1 -> Switch2/3
  brake_speed1/1 -> Switch2/1
  Bus Selector1/1 -> remap2/1(u)  "<stick_throttle>"
  Switch2/1 -> Mux1/2
  Mux1/1 -> vel_cmd_C_mPs/1

== system FMS/Control_Mode/FMS_Command_Generator/Velocity_Command/Velocity_Commander/Position_Control ==
  update : Inport
  M_CO : Inport  Port=2
  INS_Out : Inport  Port=3
  Demux : Demux  Outputs=3
  Gain1 : Gain  Gain=FMS_PARAM.XY_P  OutDataTypeStr=single
  Gain2 : Gain  Gain=FMS_PARAM.XY_P  OutDataTypeStr=single
  Gain4 : Gain  Gain=FMS_PARAM.Z_P  OutDataTypeStr=single
  Mux : Mux  Inputs=3
  Position_Error : Subsystem
  vel_cmd_C_mPs : Outport
  wires:
  INS_Out/1 -> Position_Error/2(INS_Out)
  Gain2/1 -> Mux/1
  M_CO/1 -> Position_Error/1(M_CO)
  Position_Error/1(pos_err_C_m) -> Demux/1
  Demux/1 -> Gain2/1
  Demux/2 -> Gain1/1
  Demux/3 -> Gain4/1
  Gain1/1 -> Mux/2
  Gain4/1 -> Mux/3
  Mux/1 -> vel_cmd_C_mPs/1
  update/1 -> Position_Error/3(update)

== system FMS/Control_Mode/FMS_Command_Generator/Velocity_Command/Velocity_Commander/TD ==
  v : Inport
  Integrator : DiscreteIntegrator  SampleTime=-1  ICPrevOutput=DiscIntNeverNeededParam  ICPrevScaledInput=DiscIntNeverNeededParam
  Integrator1 : DiscreteIntegrator  SampleTime=-1  ICPrevOutput=DiscIntNeverNeededParam  ICPrevScaledInput=DiscIntNeverNeededParam
  Subtract : Sum  Inputs=+-
  "fhan " : Subsystem  mask{r0=4*9.806, h0=0.05}
      mask DialogControl ParameterGroupVar Prompt: fhan(v1,v2,r0,h0)
  v1 : Outport
  wires:
  Integrator1/1 -> v1/1, Subtract/1
  v/1 -> Subtract/2
  Integrator/1 -> "fhan "/2(v2), Integrator1/1  "v2"
  Subtract/1 -> "fhan "/1(v1)
  "fhan "/1(fhan) -> Integrator/1

== system FMS/Control_Mode/FMS_Command_Generator/Psi_Rate_Command/Psi_Rate_Commander/Heading_Control/Heading_Error ==
  INS_Out : Inport
  update : Inport  Port=2
  Bus_Selection : Subsystem
  Psi_Holder : Subsystem
  Sum : Sum  Inputs=-+|
  psi_err_saturation : Subsystem
  psi_err_rad : Outport
  wires:
  Bus_Selection/1(psi_rad) -> Sum/1, Psi_Holder/1(u)  "psi_est_rad"
  update/1 -> Psi_Holder/2(update)
  INS_Out/1 -> Bus_Selection/1(INS_Out)
  Psi_Holder/1(y) -> Sum/2  "psi_cmd_rad"
  Sum/1 -> psi_err_saturation/1(psi_err_in)
  psi_err_saturation/1(psi_err_rad) -> psi_err_rad/1

== system FMS/Control_Mode/FMS_Command_Generator/Psi_Rate_Command/Psi_Rate_Commander/Motion_Heading_Rate/remap ==
  u : Inport
  Dead Zone : DeadZone  LowerValue=-th  UpperValue=th  SaturateOnIntegerOverflow=on
  Gain : Gain  Gain=1/(1-th)
  y : Outport
  wires:
  u/1 -> Dead Zone/1
  Dead Zone/1 -> Gain/1
  Gain/1 -> y/1
